simulink model "autopilot_test_harness"  (Simulink 6.0)
settings: Solver=FixedStepDiscrete  SolverMode=SingleTasking  StartTime=0.0  StopTime=300  FixedStep=0.2  RelTol=1e-3
undefined symbols (not defined in the file or in its folder): sigbuilder_block
settings Model: CovMetricSettings=dcmw  Creator=The MathWorks Inc.  LastModifiedBy=batserve  ExtModeAutoUpdateStatusClock=off  ProdHWDeviceType=Specified
settings DataIOCC: SignalLoggingName=sigsOut
settings OptimizationCC: BooleanDataType=off
settings DebuggingCC: CheckExecutionContextPreStartOutputMsg=on  CheckExecutionContextRuntimeOutputMsg=on  SolverPrmCheckMsg=none
settings HardwareCC: ProdBitPerShort=32  ProdBitPerInt=16  ProdHWDeviceType=Specified  TargetUnknown=on
settings ModelReferenceCC: UpdateModelReferenceTargets=IfOutOfDate

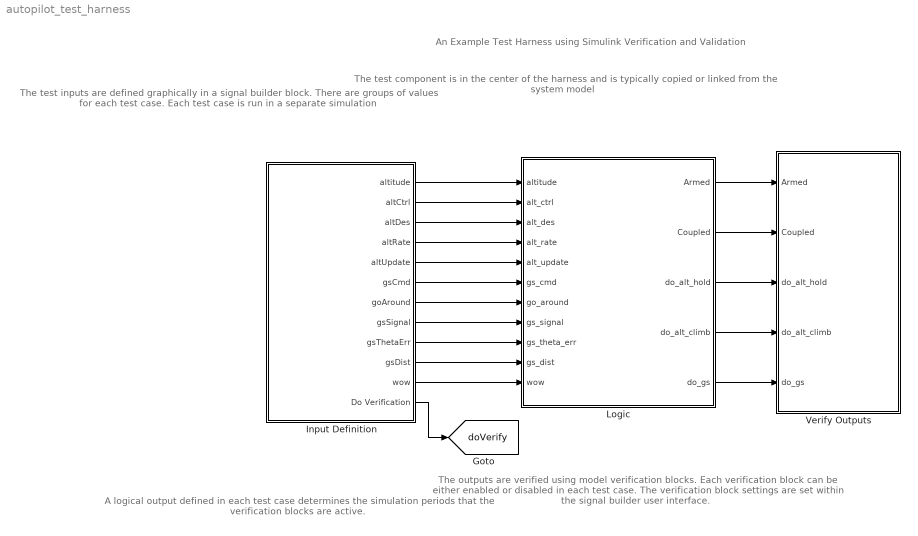
== system autopilot_test_harness ==
  note: The test inputs are defined graphically in a signal
      | builder block.  There are groups of values for each
      | test case.  Each test case is run in a separate
      | simulation
  note: The outputs are verified using model verification blocks.
      | Each verification block can be either enabled or disabled in
      | each test case.  The verification block settings are set
      | within the signal builder user interface.
  note: The test component is in the center
      | of the harness and is typically copied
      | or linked from the system model
  note: A logical output defined in each test case
      | determines the simulation periods that the
      | verification blocks are active.
  note: An Example Test Harness using Simulink Verification and Validation
  Input Definition : Subsystem  Tag=STV Subsys  RequirementInfo={ 'HTML' 'autopilot_requirements.html' 'Climb' 'true' 'Altitude Climb Control Entry Condition' '' ; 'HTML' 'autopilot_requirements.html' 'Hold' 'true' 'Altitude Hold Mode Entry Condition' '' ; 'HTML' 'autopilot_requirements.html' 'Disable' 'true' 'Autopilot Disable' '' ; 'HTML' 'autopilot_requirements.html' 'Disable' 'true' 'Autopilot Disable' '' ; 'HTML' 'autopilot_requirements.html' 'Armed' 'true' 'Glide Slope Armed Condition' '' ; 'HTML' 'autopilot_requirements.html' 'Coupled' 'true' 'Glide Slope Coupled Condition' '' }  LoadFcn=sigbuilder_block('load');  StartFcn=sigbuilder_block('start');  StopFcn=sigbuilder_block('stop');  ClipboardFcn=sigbuilder_block('clipboard');  PropExecContextAcrossSSBoundary=on  mask(Sigbuilder block){}
      mask help: Sigbuilder GUI
      mask init:
      | if ~strcmp(get_param(bdroot(gcb),'SimulationStatus'),'stopped') tuvar = sigbuilder_block('maskInit'); end
      settings: CopyFcn=sigbuilder_block('copy');  DeleteFcn=sigbuilder_block('delete');  ModelCloseFcn=sigbuilder_block('modelClose');  PreSaveFcn=sigbuilder_block('preSave');  NameChangeFcn=sigbuilder_block('namechange');  OpenFcn=sigbuilder_block('open',[21 81 593.25 412.5 ]);  CloseFcn=sigbuilder_block('close');
      mask Display: plot(0,0,100,100,[10,10,40,40,10],[80,20,20,80,80],[40,10],[50,50], [40,27,10],[65,72,56],[40,25,25,10],[28,28,43,43]);
  Logic : Stateflow chart  PropExecContextAcrossSSBoundary=on
  Verify Outputs : Subsystem  PropExecContextAcrossSSBoundary=on
  tag scope: doVerify=global
  wires:
  Input Definition/1(altitude) -> Logic/1(altitude)
  Input Definition/2(altCtrl) -> Logic/2(alt_ctrl)
  Input Definition/3(altDes) -> Logic/3(alt_des)
  Input Definition/4(altRate) -> Logic/4(alt_rate)
  Input Definition/5(altUpdate) -> Logic/5(alt_update)
  Input Definition/6(gsCmd) -> Logic/6(gs_cmd)
  Input Definition/7(goAround) -> Logic/7(go_around)
  Input Definition/8(gsSignal) -> Logic/8(gs_signal)
  Input Definition/9(gsThetaErr) -> Logic/9(gs_theta_err)
  Input Definition/10(gsDist) -> Logic/10(gs_dist)
  Input Definition/11(wow) -> Logic/11(wow)
  Logic/1(Armed) -> Verify Outputs/1(Armed)
  Logic/2(Coupled) -> Verify Outputs/2(Coupled)
  Logic/3(do_alt_hold) -> Verify Outputs/3(do_alt_hold)
  Logic/4(do_alt_climb) -> Verify Outputs/4(do_alt_climb)
  Logic/5(do_gs) -> Verify Outputs/5(do_gs)
  Input Definition/12(Do Verification) -> [doVerify]

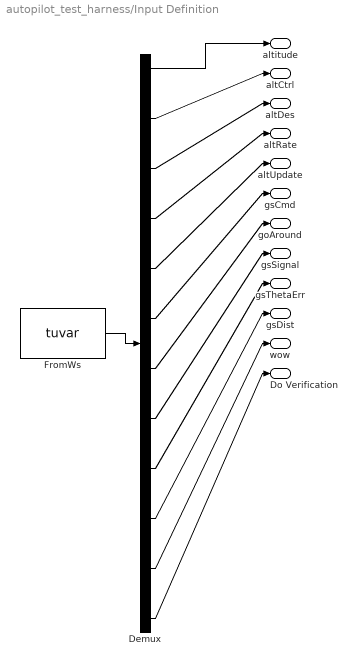
== system autopilot_test_harness/Input Definition ==
  Demux : Demux  Tag=STV Demux  Outputs=12
  FromWs : FromWorkspace  Tag=STV FromWs  VariableName=tuvar  SampleTime=0  SigBuilderData=DataTag0  VnvData=DataTag1
      SigBuilderData=|
      | channels(1).label = 'altitude'
      | channels(1).allXData = {[0 200], [0 19.5 153.5 200], [0 200], [0 200], [0 200], [0 200]}
      | channels(1).allYData = {[10000 10000], [10000 10000 12000 12000], [10000 10000], [10000 10000], [1000 1000], [1000 1000]}
      | channels(2).label = 'altCtrl'
      | channels(2).allXData = {[0 18 18 200], [0 18 18 200], [0 80.5 80.5 200], [0 80.5 80.5 200], [0 11 11 200], [0 11 11 200]}
      | channels(2).allYData = {[1 1 1 1], [1 1 1 1], [1 1 0 0], [1 1 0 0], [0 0 1 1], [0 0 1 1]}
      | channels(3).label = 'altDes'
      | channels(3).allXData = {[0 80.5 80.5 200], [0 20 20 200], [0 30.5 200], [0 30.5 30.5 200], [0 25.5 25.5 101 101 200], [0 25.5 25.5 101 101 200]}
      | channels(3).allYData = {[10000 10000 12000 12000], [10000 10000 12000 12000], [10000 10000 10000], [10000 10000 12000 12000], [1000 1000 1000 870 870 10], [1000 1000 1000 870 870 10]}
      | channels(4).label = 'altRate'
      | channels(4).allXData = {[0 83.5 83.5 200], [0 83.5 83.5 200], [0 83.5 83.5 200], [0 83.5 83.5 200], [0 8 8 200], [0 8 8 200]}
      | channels(4).allYData = {[200 200 600 600], [1000 1000 1000 1000], [200 200 600 600], [200 200 600 600], [200 200 1500 1500], [200 200 1500 1500]}
      | channels(5).label = 'altUpdate'
      | channels(5).allXData = {[0 60 60 200], [0 60 60 200], [0 60 60 200], [0 60 60 200], [0 200], [0 200]}
      | channels(5).allYData = {[1 1 1 1], [1 1 1 1], [1 1 1 1], [1 1 1 1], [1 1], [1 1]}
      | channels(6).label = 'gsCmd'
      | channels(6).allXData = {[0 200], [0 200], [0 200], [0 200], [0 5 5 200], [0 5 5 200]}
      | channels(6).allYData = {[0 0], [0 0], [0 0], [0 0], [0 0 1 1], [0 0 1 1]}
      | channels(7).label = 'goAround'
      | channels(7).allXData = {[0 200], [0 200], [0 200], [0 200], [0 200], [0 200]}
      | channels(7).allYData = {[0 0], [0 0], [0 0], [0 0], [0 0], [0 0]}
      | channels(8).label = 'gsSignal'
      | channels(8).allXData = {[0 200], [0 200], [0 200], [0 200], [0 20.5 20.5 200], [0 20.5 20.5 200]}
      | channels(8).allYData = {[0 0], [0 0], [0 0], [0 0], [0 0 1 1], [0 0 1 1]}
      | channels(9).label = 'gsThetaErr'
      | channels(9).allXData = {[0 200], [0 200], [0 200], [0 200], [0 200], [0 200]}
      | channels(9).allYData = {[0 0], [0 0], [0 0], [0 0], [-0.4 -0.4], [-0.22 0.58]}
      | channels(10).label = 'gsDist'
      | channels(10).allXData = {[0 200], [0 200], [0 200], [0 200], [0 200], [0 200]}
      | channels(10).allYData = {[0 0], [0 0], [0 0], [0 0], [11000 11000], [8000 8000]}
      | channels(11).label = 'wow'
      | channels(11).allXData = {[0 200], [0 200], [0 200], [0 200], [0 200], [0 200]}
      | channels(11).allYData = {[0 0], [0 0], [0 0], [0 0], [0 0], [0 0]}
      | channels(12).label = 'Do Verification'
      | channels(12).allXData = {[0 81 81 191 191 200], [0 150.5 150.5 198 198 200], [0 81 81 193 193 200], [0 81.5 81.5 191 191 200], [0 60 60 193.5 193.5 200], [0 80 80 193.5 193.5 200]}
      | channels(12).allYData = {[0 0 1 1 0 0], [0 0 1 1 0 0], [0 0 1 1 0 0], [0 0 1 1 0 0], [0 0 1 1 0 0], [0 0 1 1 0 0]}
      | dataSet(1).timeRange = [0 200]
      | dataSet(1).name = 'Enter climb mode'
      | dataSet(2).timeRange = [0 200]
      | dataSet(2).name = 'Transition to hold mode'
      | dataSet(3).timeRange = [0 200]
      | dataSet(3).name = 'Control disable (hold)'
      | dataSet(4).timeRange = [0 200]
      | dataSet(4).name = 'Control disable (climb)'
      | dataSet(5).timeRange = [0 200]
      | dataSet(5).name = 'Glideslope armed'
      | dataSet(6).timeRange = [0 200]
      | dataSet(6).name = 'Glideslope coupled'
  altitude : Outport  Tag=STV Outport
  altCtrl : Outport  Tag=STV Outport  Port=2
  altDes : Outport  Tag=STV Outport  Port=3
  altRate : Outport  Tag=STV Outport  Port=4
  altUpdate : Outport  Tag=STV Outport  Port=5
  gsCmd : Outport  Tag=STV Outport  Port=6
  goAround : Outport  Tag=STV Outport  Port=7
  gsSignal : Outport  Tag=STV Outport  Port=8
  gsThetaErr : Outport  Tag=STV Outport  Port=9
  gsDist : Outport  Tag=STV Outport  Port=10
  wow : Outport  Tag=STV Outport  Port=11
  Do Verification : Outport  Tag=STV Outport  Port=12
  wires:
  Demux/1 -> altitude/1
  FromWs/1 -> Demux/1
  Demux/2 -> altCtrl/1
  Demux/3 -> altDes/1
  Demux/4 -> altRate/1
  Demux/5 -> altUpdate/1
  Demux/6 -> gsCmd/1
  Demux/7 -> goAround/1
  Demux/8 -> gsSignal/1
  Demux/9 -> gsThetaErr/1
  Demux/10 -> gsDist/1
  Demux/11 -> wow/1
  Demux/12 -> Do Verification/1

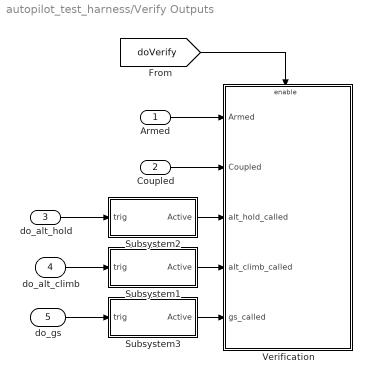
== system autopilot_test_harness/Verify Outputs ==
  Armed : Inport  Port=1  LatchInput=off
  Coupled : Inport  Port=2  LatchInput=off
  do_alt_hold : Inport  Port=3  LatchInput=off
  do_alt_climb : Inport  Port=4  LatchInput=off
  do_gs : Inport  Port=5  LatchInput=off
  Subsystem1 : Subsystem  PropExecContextAcrossSSBoundary=on
      mask Display: disp('Is Active')
  Subsystem2 : Subsystem  PropExecContextAcrossSSBoundary=on
      mask Display: disp('Is Active')
  Subsystem3 : Subsystem  PropExecContextAcrossSSBoundary=on
      mask Display: disp('Is Active')
  Verification : Subsystem  PropExecContextAcrossSSBoundary=on
  wires:
  Armed/1 -> Verification/1(Armed)
  Coupled/1 -> Verification/2(Coupled)
  do_gs/1 -> Subsystem3/1(trig)
  Subsystem2/1(Active) -> Verification/3(alt_hold_called)
  Subsystem1/1(Active) -> Verification/4(alt_climb_called)
  Subsystem3/1(Active) -> Verification/5(gs_called)
  [doVerify] -> Verification/Enable
  do_alt_climb/1 -> Subsystem1/1(trig)
  do_alt_hold/1 -> Subsystem2/1(trig)

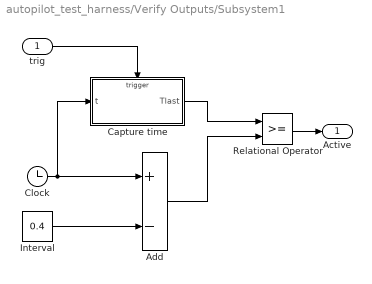
== system autopilot_test_harness/Verify Outputs/Subsystem1 ==
  trig : Inport  Port=1  LatchInput=off
  Add : Sum  Inputs=+-  OutScaling=2^-10
  Capture time : Subsystem  TreatAsAtomicUnit=on  PropExecContextAcrossSSBoundary=on
  Clock : Clock
      settings: Decimation=10
  Interval : Constant  Value=0.4
  Relational Operator : RelationalOperator  LogicOutDataTypeMode=Boolean
  Active : Outport
  wires:
  trig/1 -> Capture time/Trigger
  Add/1 -> Relational Operator/2
  Relational Operator/1 -> Active/1
  Interval/1 -> Add/2
  Clock/1 -> Capture time/1(t), Add/1
  Capture time/1(Tlast) -> Relational Operator/1

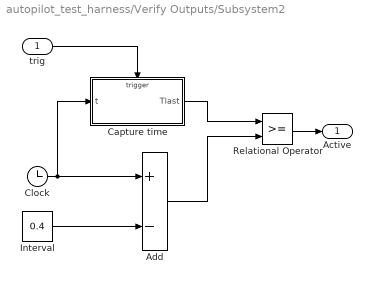
== system autopilot_test_harness/Verify Outputs/Subsystem2 ==
  trig : Inport  Port=1  LatchInput=off
  Add : Sum  Inputs=+-  OutScaling=2^-10
  Capture time : Subsystem  TreatAsAtomicUnit=on  PropExecContextAcrossSSBoundary=on
  Clock : Clock
      settings: Decimation=10
  Interval : Constant  Value=0.4
  Relational Operator : RelationalOperator  LogicOutDataTypeMode=Boolean
  Active : Outport
  wires:
  Capture time/1(Tlast) -> Relational Operator/1
  Clock/1 -> Add/1, Capture time/1(t)
  Interval/1 -> Add/2
  Relational Operator/1 -> Active/1
  Add/1 -> Relational Operator/2
  trig/1 -> Capture time/Trigger

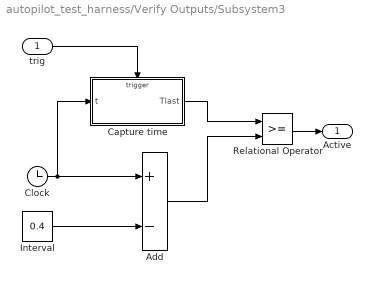
== system autopilot_test_harness/Verify Outputs/Subsystem3 ==
  trig : Inport  Port=1  LatchInput=off
  Add : Sum  Inputs=+-  OutScaling=2^-10
  Capture time : Subsystem  TreatAsAtomicUnit=on  PropExecContextAcrossSSBoundary=on
  Clock : Clock
      settings: Decimation=10
  Interval : Constant  Value=0.4
  Relational Operator : RelationalOperator  LogicOutDataTypeMode=Boolean
  Active : Outport
  wires:
  Capture time/1(Tlast) -> Relational Operator/1
  Clock/1 -> Add/1, Capture time/1(t)
  Interval/1 -> Add/2
  Relational Operator/1 -> Active/1
  Add/1 -> Relational Operator/2
  trig/1 -> Capture time/Trigger

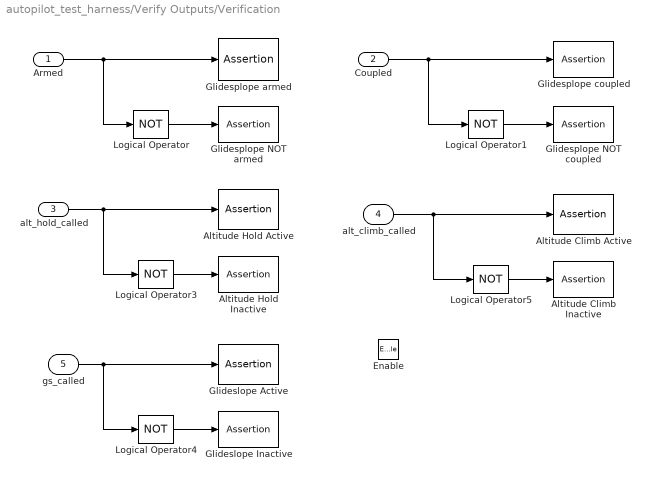
== system autopilot_test_harness/Verify Outputs/Verification ==
  Armed : Inport  Port=1  LatchInput=off
  Coupled : Inport  Port=2  LatchInput=off
  alt_hold_called : Inport  Port=3  LatchInput=off
  alt_climb_called : Inport  Port=4  LatchInput=off
  gs_called : Inport  Port=5  LatchInput=off
  Enable : EnablePort
  Altitude Climb Active : Assertion  Enabled=off  StopWhenAssertionFail=off
  Altitude Climb Inactive : Assertion  Enabled=off
  Altitude Hold Active : Assertion  Enabled=off
  Altitude Hold Inactive : Assertion  Enabled=off
  Glideslope Active : Assertion  Enabled=off
  Glideslope Inactive : Assertion  Enabled=off
  Glidesplope NOT armed : Assertion  Enabled=off
  Glidesplope NOT coupled : Assertion  Enabled=off
  Glidesplope armed : Assertion  Enabled=off
  Glidesplope coupled : Assertion  Enabled=off
  Logical Operator{,1,3..5} (5 alike) : Logic  Operator=NOT  AllPortsSameDT=off  OutDataTypeMode=Boolean
  wires:
  Armed/1 -> Glidesplope armed/1, Logical Operator/1
  Coupled/1 -> Glidesplope coupled/1, Logical Operator1/1
  Logical Operator/1 -> Glidesplope NOT armed/1
  Logical Operator1/1 -> Glidesplope NOT coupled/1
  alt_hold_called/1 -> Logical Operator3/1, Altitude Hold Active/1
  Logical Operator3/1 -> Altitude Hold Inactive/1
  gs_called/1 -> Logical Operator4/1, Glideslope Active/1
  Logical Operator4/1 -> Glideslope Inactive/1
  alt_climb_called/1 -> Logical Operator5/1, Altitude Climb Active/1
  Logical Operator5/1 -> Altitude Climb Inactive/1

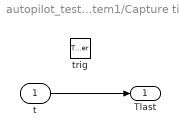
== system autopilot_test_harness/Verify Outputs/Subsystem1/Capture time ==
  t : Inport  Port=1  LatchInput=off
  trig : TriggerPort  TriggerType=function-call  ZeroCross=off
  Tlast : Outport  InitialOutput=-999
  wires:
  t/1 -> Tlast/1

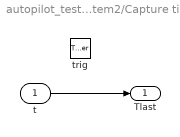
== system autopilot_test_harness/Verify Outputs/Subsystem2/Capture time ==
  t : Inport  Port=1  LatchInput=off
  trig : TriggerPort  TriggerType=function-call  ZeroCross=off
  Tlast : Outport  InitialOutput=-999
  wires:
  t/1 -> Tlast/1

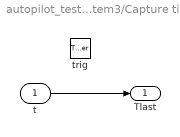
== system autopilot_test_harness/Verify Outputs/Subsystem3/Capture time ==
  t : Inport  Port=1  LatchInput=off
  trig : TriggerPort  TriggerType=function-call  ZeroCross=off
  Tlast : Outport  InitialOutput=-999
  wires:
  t/1 -> Tlast/1

== stateflow chart Logic ==
  settings: updateMethod=DISCRETE  sampleTime=0.2
  state out = alt_capture() [function]
    (default) -> (junction 19) : {out = abs(altitude - alt_des) < 30*ts*(alt_rate / 60);}
  state GS [parallel]
    state Off
    state Active
      state Armed
      state Coupled /du: do_gs;
        state Around
        state Norm
        (default) -> Norm
        Norm -> Around : [go_around]
      Armed -> Coupled /du: do_gs; : [gs_coupled()]
      (default) -> Armed
    GS.Active -> Off : [~gs_cmd | ...
        |  ~gs_signal | wow]
    (default) -> Off
    Off -> GS.Active : [gs_cmd & ...
        | gs_signal & ~wow]
  state out = gs_coupled() [function]
    (default) -> (junction 18) : {out = gs_dist<10000 & gs_theta_err>0;}
  note: Glideslope
  state Altitude [parallel]
    state Disabled
    state Active
      state Climb_Rate
        du: do_alt_climb;
      state Hold
        du: do_alt_hold;
      Hold -> Climb_Rate : [abs(altitude-alt_des) >1500]
      Climb_Rate -> Hold : [alt_capture()]
    Disabled -> Hold : [alt_ctrl & ~wow & ...
        | ~in(GS.Active.Coupled)]
    (default) -> Disabled
    Altitude.Active -> Disabled : [in(GS.Active.Coupled) | ...
        | ~alt_ctrl | wow]
  data: out function_output double size=1; out function_output double size=1; altitude input double size=1; alt_ctrl input double size=1; alt_des input double size=1; alt_rate input double size=1; alt_update input double size=1; gs_cmd input double size=1; go_around input double size=1; gs_signal input double size=1; gs_theta_err input double size=1; gs_dist input double size=1; ts constant double size=1 =0.2; Armed output State size=1; Coupled output State size=1; wow input double size=1
  events: do_alt_hold output FUNCTION_CALL_EVENT; do_alt_climb output FUNCTION_CALL_EVENT; do_gs output FUNCTION_CALL_EVENT
